simulink model "IMU_Simulation"  (Simulink 7.9)
settings: Solver=FixedStepDiscrete  StartTime=0.0  StopTime=25  FixedStep=.001  RelTol=1e-3
PreLoadFcn:
  | Script_Kalman
values from neighbouring files (symbols this model uses):
  Az = [1 -Ts ;0 1]    [Script_Kalman.m]
  Kz = 1e-3*[.4 ; -.04]    [Script_Kalman.m]
  Ts = .001    (= 0.001)    [Script_Kalman.m]
undefined symbols (not defined in the file or in its folder): dend, DiscIntNeverNeededParam, gaind, numd, polesd, zerosd
libraries: simulink x38
(part 1 of 2)
settings Model: Creator=Lubin  LastModifiedBy=denis.pretre
settings OptimizationCC: InitFltsAndDblsToZero=on
settings DebuggingCC: MultiTaskCondExecSysMsg=warning  MultiTaskRateTransMsg=warning  FcnCallInpInsideContextMsg=Use local settings  StrictBusMsg=Warning
settings HardwareCC: TargetHWDeviceType=32-bit Generic
settings GRTTargetCC: TargetFcnLib=ansi_tfl_tmw.mat  CombineOutputUpdateFcns=off  GRTInterface=on

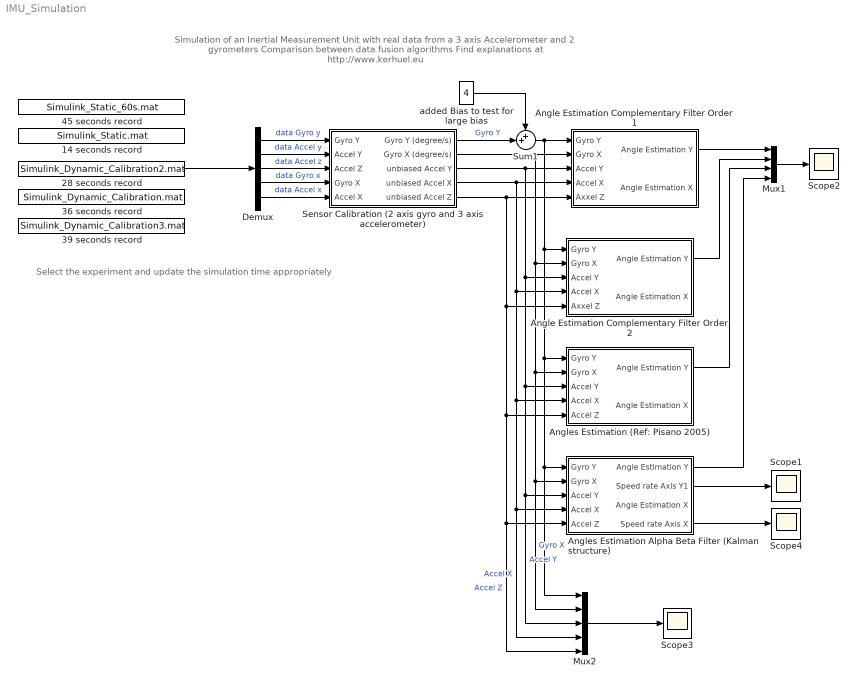
== system IMU_Simulation ==
  note: Simulation of an Inertial Measurement Unit with real data from a 3 axis Accelerometer and 2 gyrometers
      | Comparison between data fusion algorithms
      | Find explanations at http://www.kerhuel.eu
  note: Select the experiment and
      | update the simulation time appropriately
  14 seconds record : FromFile  FileName=Simulink_Static.mat  SampleTime=.001
  28 seconds record : FromFile  FileName=Simulink_Dynamic_Calibration2.mat  SampleTime=.001
  36 seconds record : FromFile  FileName=Simulink_Dynamic_Calibration.mat  SampleTime=.001
  39 seconds record : FromFile  FileName=Simulink_Dynamic_Calibration3.mat  SampleTime=.001
  45 seconds record : FromFile  FileName=Simulink_Static_60s.mat  SampleTime=.001
  Angle Estimation Complementary Filter Order 1 : Subsystem
  Angle Estimation Complementary Filter Order 2 : Subsystem
  Angles Estimation (Ref: Pisano 2005) : Subsystem
  Angles Estimation Alpha Beta Filter (Kalman structure) : Subsystem
  Demux : Demux  Outputs=5
  Mux1 : Mux
  Mux2 : Mux  Inputs=5
  Scope{1..4} (4 alike) : Scope
      Scope1 settings: TimeRange=9.424342105263159  YMin=-7  YMax=7  SaveName=ScopeData3
      Scope2 settings: TickLabels=on  ShowLegends=on  TimeRange=30  YMin=0.5  YMax=10  SaveName=ScopeData4  MaxDataPoints=50000  Decimation=10
      Scope3 settings: TickLabels=on  ShowLegends=on  TimeRange=30  YMin=0.5  YMax=10  SaveName=ScopeData5  MaxDataPoints=50000  Decimation=10
      Scope4 settings: TimeRange=9.424342105263159  YMin=-1.75  YMax=1.75  SaveName=ScopeData6
  Sensor Calibration (2 axis gyro and 3 axis accelerometer) : Subsystem
  Sum1 : Sum  Inputs=++|
  added Bias to test for large bias : Constant  Value=4
  wires:
  Demux/2 -> Sensor Calibration (2 axis gyro and 3 axis accelerometer)/2(Accel Y)  "data Accel y"
  Demux/3 -> Sensor Calibration (2 axis gyro and 3 axis accelerometer)/3(Accel Z)  "data Accel z"
  Demux/4 -> Sensor Calibration (2 axis gyro and 3 axis accelerometer)/4(Gyro X)  "data Gyro x"
  Demux/5 -> Sensor Calibration (2 axis gyro and 3 axis accelerometer)/5(Accel X)  "data Accel x"
  Demux/1 -> Sensor Calibration (2 axis gyro and 3 axis accelerometer)/1(Gyro Y)  "data Gyro y"
  Sensor Calibration (2 axis gyro and 3 axis accelerometer)/1(Gyro Y (degree/s)) -> Sum1/2  "Gyro Y"
  Sensor Calibration (2 axis gyro and 3 axis accelerometer)/2(Gyro X (degree/s)) -> Angle Estimation Complementary Filter Order 1/2(Gyro X), Angles Estimation (Ref: Pisano 2005)/2(Gyro X), Angles Estimation Alpha Beta Filter (Kalman structure)/2(Gyro X), Mux2/2, Angle Estimation Complementary Filter Order 2/2(Gyro X)  "Gyro X"
  Sensor Calibration (2 axis gyro and 3 axis accelerometer)/3(unbiased Accel Y) -> Angle Estimation Complementary Filter Order 1/3(Accel Y), Angles Estimation (Ref: Pisano 2005)/3(Accel Y), Angles Estimation Alpha Beta Filter (Kalman structure)/3(Accel Y), Mux2/3, Angle Estimation Complementary Filter Order 2/3(Accel Y)  "Accel Y"
  Sensor Calibration (2 axis gyro and 3 axis accelerometer)/4(unbiased Accel X) -> Angle Estimation Complementary Filter Order 1/4(Accel X), Angles Estimation (Ref: Pisano 2005)/4(Accel X), Angles Estimation Alpha Beta Filter (Kalman structure)/4(Accel X), Mux2/4, Angle Estimation Complementary Filter Order 2/4(Accel X)  "Accel X"
  Sensor Calibration (2 axis gyro and 3 axis accelerometer)/5(unbiased Accel Z) -> Angle Estimation Complementary Filter Order 1/5(Axxel Z), Angles Estimation (Ref: Pisano 2005)/5(Accel Z), Angles Estimation Alpha Beta Filter (Kalman structure)/5(Accel Z), Mux2/5, Angle Estimation Complementary Filter Order 2/5(Axxel Z)  "Accel Z"
  Mux1/1 -> Scope2/1
  Angle Estimation Complementary Filter Order 1/1(Angle Estimation Y) -> Mux1/1
  Angle Estimation Complementary Filter Order 2/1(Angle Estimation Y) -> Mux1/2
  Angles Estimation (Ref: Pisano 2005)/1(Angle Estimation Y) -> Mux1/3
  Angles Estimation Alpha Beta Filter (Kalman structure)/1(Angle Estimation Y) -> Mux1/4
  Sum1/1 -> Angle Estimation Complementary Filter Order 1/1("Gyro Y "), Angles Estimation (Ref: Pisano 2005)/1(Gyro Y), Angles Estimation Alpha Beta Filter (Kalman structure)/1(Gyro Y), Mux2/1, Angle Estimation Complementary Filter Order 2/1("Gyro Y ")
  added Bias to test for large bias/1 -> Sum1/1
  Angles Estimation Alpha Beta Filter (Kalman structure)/2(Speed rate Axis Y1) -> Scope1/1
  Angles Estimation Alpha Beta Filter (Kalman structure)/4(Speed rate Axis X) -> Scope4/1
  28 seconds record/1 -> Demux/1
  Mux2/1 -> Scope3/1

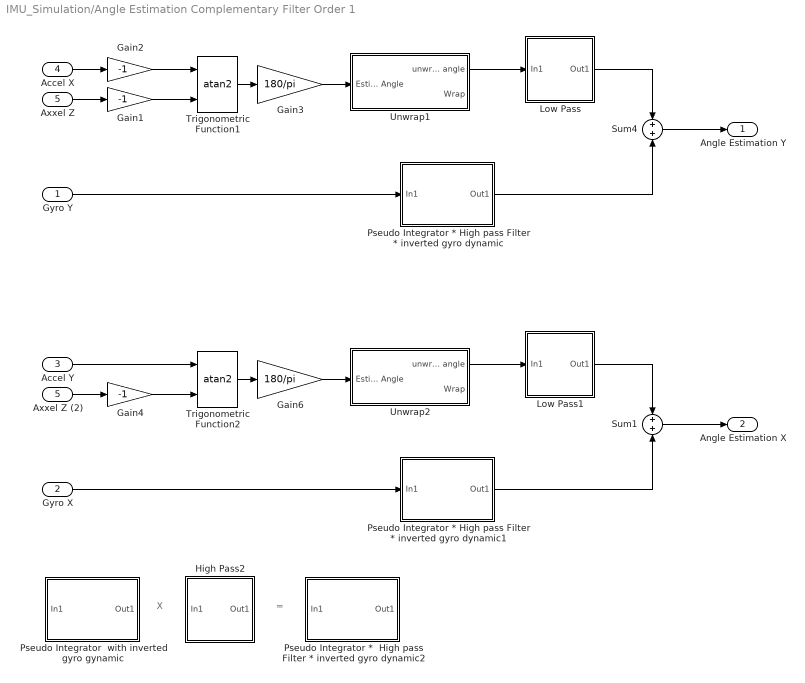
== system IMU_Simulation/Angle Estimation Complementary Filter Order 1 ==
  note: X
  note: =
  "Gyro Y " : Inport
  Gyro X : Inport  Port=2
  Accel Y : Inport  Port=3
  Accel X : Inport  Port=4
  Axxel Z : Inport  Port=5
  Axxel Z (2) : InportShadow  Port=5
  Gain1 : Gain  Gain=-1
  Gain2 : Gain  Gain=-1
  Gain3 : Gain  Gain=180/pi  OutDataTypeStr=float('double')
  Gain4 : Gain  Gain=-1
  Gain6 : Gain  Gain=180/pi  OutDataTypeStr=float('double')
  High Pass2 : Subsystem  mask(DiscretizedZeroPole){Zeros=[0], Poles=[-.5], Gain=1, AbsTol=auto, SampleTime=.001, method=tustin, Wc=1}
      mask prompts: Zeros "Zeros (enter in s-main:)"; Poles "Poles (enter in s-domain:)"; Gain "Gain (enter in s-domain:)"; AbsTol "Absolute tolerance:"; SampleTime "Sample time:"; Wc "Critical Frequency (Hz):"
      mask help: Continuous mask uses c2d to transform parameters onto the Discrete Zero-Pole block inside.
      mask init:
      | st=SampleTime;
      | if length(st)>1
      |     st=SampleTime(1);
      | end
      | if(st>0)
      |     [zerosd,polesd,gaind] = sldiscutil('disczpk', {st,method,Wc,Zeros,Poles,Gain});
      | end	
      | s = get_param(gcb,'maskvalues');
      | zeross = s{1};
      | poless = s{2};
      | gainss = s{3};
      | %zerosc = eval(zeross);
      | %polesc = eval(poless);
      | %gainsc = eval(gainss);
      | sldiscutil('initzpkmask', st);
      | if(st==0)
      | set_param([gcb '/Zero Pole'], 'AbsoluteTolerance', AbsTol);
      | end
      mask StyleString: edit,edit,edit,edit,edit,popup(zoh|foh|tustin|prewarp|matched),edit
      mask CallbackString: |||||hidecrit|
      mask Display:
      | droots(zeross,poless,gainss)
      | text( 0.5, 1.0, method, 'verticalAlignment','top')
  Low Pass : Subsystem  mask(DiscretizedZeroPole){Zeros=[], Poles=[-.5], Gain=.5, AbsTol=auto, SampleTime=.001, method=tustin, Wc=1}
      mask prompts: Zeros "Zeros (enter in s-main:)"; Poles "Poles (enter in s-domain:)"; Gain "Gain (enter in s-domain:)"; AbsTol "Absolute tolerance:"; SampleTime "Sample time:"; Wc "Critical Frequency (Hz):"
      mask help: Continuous mask uses c2d to transform parameters onto the Discrete Zero-Pole block inside.
      mask init: same as IMU_Simulation/Angle Estimation Complementary Filter Order 1/High Pass2
      mask StyleString: edit,edit,edit,edit,edit,popup(zoh|foh|tustin|prewarp|matched),edit
      mask CallbackString: |||||hidecrit|
      mask Display:
      | droots(zeross,poless,gainss)
      | text( 0.5, 1.0, method, 'verticalAlignment','top')
  Low Pass1 : Subsystem  mask(DiscretizedZeroPole){Zeros=[], Poles=[-.5], Gain=.5, AbsTol=auto, SampleTime=.001, method=tustin, Wc=1}
      mask prompts: Zeros "Zeros (enter in s-main:)"; Poles "Poles (enter in s-domain:)"; Gain "Gain (enter in s-domain:)"; AbsTol "Absolute tolerance:"; SampleTime "Sample time:"; Wc "Critical Frequency (Hz):"
      mask help: Continuous mask uses c2d to transform parameters onto the Discrete Zero-Pole block inside.
      mask init: same as IMU_Simulation/Angle Estimation Complementary Filter Order 1/High Pass2
      mask StyleString: edit,edit,edit,edit,edit,popup(zoh|foh|tustin|prewarp|matched),edit
      mask CallbackString: |||||hidecrit|
      mask Display:
      | droots(zeross,poless,gainss)
      | text( 0.5, 1.0, method, 'verticalAlignment','top')
  Pseudo Integrator  with inverted gyro gynamic : Subsystem  mask(DiscretizedZeroPole){Zeros=[-314], Poles=[0], Gain=(1/314), AbsTol=auto, SampleTime=.001, method=tustin, Wc=1}
      mask prompts: Zeros "Zeros (enter in s-main:)"; Poles "Poles (enter in s-domain:)"; Gain "Gain (enter in s-domain:)"; AbsTol "Absolute tolerance:"; SampleTime "Sample time:"; Wc "Critical Frequency (Hz):"
      mask help: Continuous mask uses c2d to transform parameters onto the Discrete Zero-Pole block inside.
      mask init: same as IMU_Simulation/Angle Estimation Complementary Filter Order 1/High Pass2
      mask StyleString: edit,edit,edit,edit,edit,popup(zoh|foh|tustin|prewarp|matched),edit
      mask CallbackString: |||||hidecrit|
      mask Display:
      | droots(zeross,poless,gainss)
      | text( 0.5, 1.0, method, 'verticalAlignment','top')
  Pseudo Integrator *  High pass Filter * inverted gyro dynamic2 : Subsystem  mask(DiscretizedZeroPole){Zeros=[-314], Poles=[-.5], Gain=(1/314), AbsTol=auto, SampleTime=.001, method=tustin, Wc=1}
      mask prompts: Zeros "Zeros (enter in s-main:)"; Poles "Poles (enter in s-domain:)"; Gain "Gain (enter in s-domain:)"; AbsTol "Absolute tolerance:"; SampleTime "Sample time:"; Wc "Critical Frequency (Hz):"
      mask help: Continuous mask uses c2d to transform parameters onto the Discrete Zero-Pole block inside.
      mask init: same as IMU_Simulation/Angle Estimation Complementary Filter Order 1/High Pass2
      mask StyleString: edit,edit,edit,edit,edit,popup(zoh|foh|tustin|prewarp|matched),edit
      mask CallbackString: |||||hidecrit|
      mask Display:
      | droots(zeross,poless,gainss)
      | text( 0.5, 1.0, method, 'verticalAlignment','top')
  Pseudo Integrator * High pass Filter * inverted gyro dynamic : Subsystem  mask(DiscretizedZeroPole){Zeros=[-314], Poles=[-.5], Gain=(1/314), AbsTol=auto, SampleTime=.001, method=tustin, Wc=1}
      mask prompts: Zeros "Zeros (enter in s-main:)"; Poles "Poles (enter in s-domain:)"; Gain "Gain (enter in s-domain:)"; AbsTol "Absolute tolerance:"; SampleTime "Sample time:"; Wc "Critical Frequency (Hz):"
      mask help: Continuous mask uses c2d to transform parameters onto the Discrete Zero-Pole block inside.
      mask init: same as IMU_Simulation/Angle Estimation Complementary Filter Order 1/High Pass2
      mask StyleString: edit,edit,edit,edit,edit,popup(zoh|foh|tustin|prewarp|matched),edit
      mask CallbackString: |||||hidecrit|
      mask Display:
      | droots(zeross,poless,gainss)
      | text( 0.5, 1.0, method, 'verticalAlignment','top')
  Pseudo Integrator * High pass Filter * inverted gyro dynamic1 : Subsystem  mask(DiscretizedZeroPole){Zeros=[-314], Poles=[-.5], Gain=(1/314), AbsTol=auto, SampleTime=.001, method=tustin, Wc=1}
      mask prompts: Zeros "Zeros (enter in s-main:)"; Poles "Poles (enter in s-domain:)"; Gain "Gain (enter in s-domain:)"; AbsTol "Absolute tolerance:"; SampleTime "Sample time:"; Wc "Critical Frequency (Hz):"
      mask help: Continuous mask uses c2d to transform parameters onto the Discrete Zero-Pole block inside.
      mask init: same as IMU_Simulation/Angle Estimation Complementary Filter Order 1/High Pass2
      mask StyleString: edit,edit,edit,edit,edit,popup(zoh|foh|tustin|prewarp|matched),edit
      mask CallbackString: |||||hidecrit|
      mask Display:
      | droots(zeross,poless,gainss)
      | text( 0.5, 1.0, method, 'verticalAlignment','top')
  Sum1 : Sum  SaturateOnIntegerOverflow=on
  Sum4 : Sum  SaturateOnIntegerOverflow=on
  Trigonometric Function1 : Trigonometry  Operator=atan2  OutputSignalType=real
  Trigonometric Function2 : Trigonometry  Operator=atan2  OutputSignalType=real
  Unwrap1 : Subsystem
  Unwrap2 : Subsystem
  Angle Estimation Y : Outport
  Angle Estimation X : Outport  Port=2
  wires:
  Unwrap2/1(unwrap angle) -> Low Pass1/1(In1)
  Gain6/1 -> Unwrap2/1(Estimated Angle)
  Trigonometric Function2/1 -> Gain6/1
  Gain4/1 -> Trigonometric Function2/2
  Gyro X/1 -> Pseudo Integrator * High pass Filter * inverted gyro dynamic1/1(In1)
  Sum1/1 -> Angle Estimation X/1
  Axxel Z (2)/1 -> Gain4/1
  Accel Y/1 -> Trigonometric Function2/1
  Low Pass1/1(Out1) -> Sum1/1
  Unwrap1/1(unwrap angle) -> Low Pass/1(In1)
  Gain3/1 -> Unwrap1/1(Estimated Angle)
  Trigonometric Function1/1 -> Gain3/1
  Gain1/1 -> Trigonometric Function1/2
  Gain2/1 -> Trigonometric Function1/1
  "Gyro Y "/1 -> Pseudo Integrator * High pass Filter * inverted gyro dynamic/1(In1)
  Sum4/1 -> Angle Estimation Y/1
  Axxel Z/1 -> Gain1/1
  Accel X/1 -> Gain2/1
  Low Pass/1(Out1) -> Sum4/1
  Pseudo Integrator * High pass Filter * inverted gyro dynamic1/1(Out1) -> Sum1/2
  Pseudo Integrator * High pass Filter * inverted gyro dynamic/1(Out1) -> Sum4/2

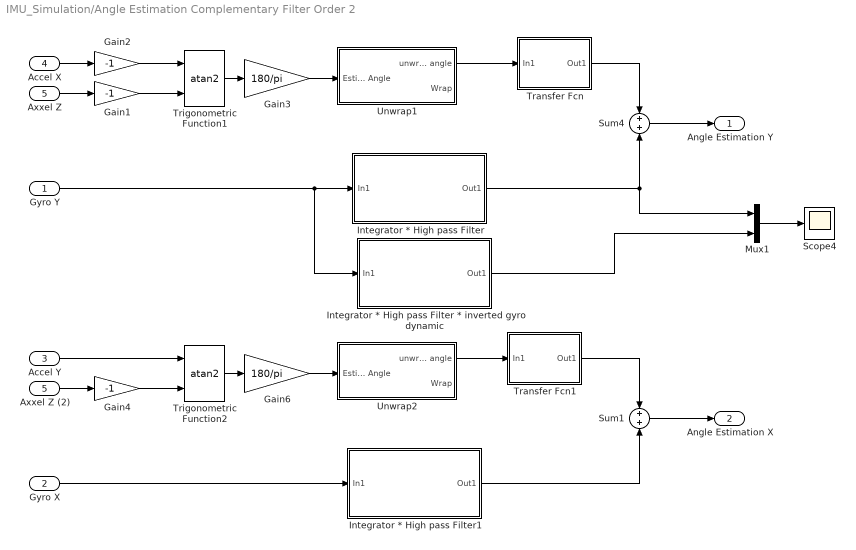
== system IMU_Simulation/Angle Estimation Complementary Filter Order 2 ==
  "Gyro Y " : Inport
  Gyro X : Inport  Port=2
  Accel Y : Inport  Port=3
  Accel X : Inport  Port=4
  Axxel Z : Inport  Port=5
  Axxel Z (2) : InportShadow  Port=5
  Gain1 : Gain  Gain=-1
  Gain2 : Gain  Gain=-1
  Gain3 : Gain  Gain=180/pi  OutDataTypeStr=float('double')
  Gain4 : Gain  Gain=-1
  Gain6 : Gain  Gain=180/pi  OutDataTypeStr=float('double')
  Integrator * High pass Filter : Subsystem  mask(DiscretizedZeroPole){Zeros=[0], Poles=[-.2 -.2], Gain=1, AbsTol=auto, SampleTime=.001, method=tustin, Wc=1}
      mask prompts: Zeros "Zeros (enter in s-main:)"; Poles "Poles (enter in s-domain:)"; Gain "Gain (enter in s-domain:)"; AbsTol "Absolute tolerance:"; SampleTime "Sample time:"; Wc "Critical Frequency (Hz):"
      mask help: Continuous mask uses c2d to transform parameters onto the Discrete Zero-Pole block inside.
      mask init: same as IMU_Simulation/Angle Estimation Complementary Filter Order 1/High Pass2
      mask StyleString: edit,edit,edit,edit,edit,popup(zoh|foh|tustin|prewarp|matched),edit
      mask CallbackString: |||||hidecrit|
      mask Display:
      | droots(zeross,poless,gainss)
      | text( 0.5, 1.0, method, 'verticalAlignment','top')
  Integrator * High pass Filter * inverted gyro dynamic : Subsystem  mask(DiscretizedZeroPole){Zeros=[-314 0], Poles=[-.2 -.2], Gain=(1/314), AbsTol=auto, SampleTime=.001, method=tustin, Wc=1}
      mask prompts: Zeros "Zeros (enter in s-main:)"; Poles "Poles (enter in s-domain:)"; Gain "Gain (enter in s-domain:)"; AbsTol "Absolute tolerance:"; SampleTime "Sample time:"; Wc "Critical Frequency (Hz):"
      mask help: Continuous mask uses c2d to transform parameters onto the Discrete Zero-Pole block inside.
      mask init: same as IMU_Simulation/Angle Estimation Complementary Filter Order 1/High Pass2
      mask StyleString: edit,edit,edit,edit,edit,popup(zoh|foh|tustin|prewarp|matched),edit
      mask CallbackString: |||||hidecrit|
      mask Display:
      | droots(zeross,poless,gainss)
      | text( 0.5, 1.0, method, 'verticalAlignment','top')
  Integrator * High pass Filter1 : Subsystem  mask(DiscretizedZeroPole){Zeros=[0], Poles=[-.2 -.2], Gain=1, AbsTol=auto, SampleTime=.001, method=tustin, Wc=1}
      mask prompts: Zeros "Zeros (enter in s-main:)"; Poles "Poles (enter in s-domain:)"; Gain "Gain (enter in s-domain:)"; AbsTol "Absolute tolerance:"; SampleTime "Sample time:"; Wc "Critical Frequency (Hz):"
      mask help: Continuous mask uses c2d to transform parameters onto the Discrete Zero-Pole block inside.
      mask init: same as IMU_Simulation/Angle Estimation Complementary Filter Order 1/High Pass2
      mask StyleString: edit,edit,edit,edit,edit,popup(zoh|foh|tustin|prewarp|matched),edit
      mask CallbackString: |||||hidecrit|
      mask Display:
      | droots(zeross,poless,gainss)
      | text( 0.5, 1.0, method, 'verticalAlignment','top')
  Mux1 : Mux  Inputs=2
  Scope4 : Scope
      settings: TimeRange=9.424342105263159  YMin=0.5  YMax=6.25  SaveName=ScopeData2  Decimation=10
  Sum1 : Sum  SaturateOnIntegerOverflow=on
  Sum4 : Sum  SaturateOnIntegerOverflow=on
  Transfer Fcn : Subsystem  mask(DiscretizedTransferFcn){Numerator=[.4 .02], Denominator=[1 .4 .02], AbsTol=auto, SampleTime=.001, method=tustin, Wc=0}
      mask prompts: Numerator "Numerator (enter in s-domain:)"; Denominator "Denominator (enter in s-domain:)"; AbsTol "Absolute tolerance:"; SampleTime "Sample time:"; Wc "Critical Frequency (Hz):"
      mask help: Continuous mask uses c2d to transform parameters onto the Discrete Transfer function block inside.
      mask init:
      | st=SampleTime;
      | if length(st)>1
      |     st=SampleTime(1);
      | end
      | if(st>0)
      |     [numd,dend] = sldiscutil('disctransferfcn',{st,method,Wc,Numerator,Denominator});
      | end	
      | s = get_param(gcb,'maskvalues');
      | nums = s{1};
      | dens = s{2};
      | %numc = eval(nums);
      | %denc = eval(dens);
      | sldiscutil('inittfmask', st);
      | if(st==0)
      | set_param([gcb '/Transfer Fcn'], 'AbsoluteTolerance', AbsTol);
      | end
      mask StyleString: edit,edit,edit,edit,popup(zoh|foh|tustin|prewarp|matched),edit
      mask CallbackString: ||||hidecrit|
      mask Display:
      | dpoly(nums,dens)
      | text( 0.5, 1.0, method, 'verticalAlignment','top')
  Transfer Fcn1 : Subsystem  mask(DiscretizedTransferFcn){Numerator=[.4 .02], Denominator=[1 .4 .02], AbsTol=auto, SampleTime=.001, method=tustin, Wc=0}
      mask prompts: Numerator "Numerator (enter in s-domain:)"; Denominator "Denominator (enter in s-domain:)"; AbsTol "Absolute tolerance:"; SampleTime "Sample time:"; Wc "Critical Frequency (Hz):"
      mask help: Continuous mask uses c2d to transform parameters onto the Discrete Transfer function block inside.
      mask init: same as IMU_Simulation/Angle Estimation Complementary Filter Order 2/Transfer Fcn
      mask StyleString: edit,edit,edit,edit,popup(zoh|foh|tustin|prewarp|matched),edit
      mask CallbackString: ||||hidecrit|
      mask Display:
      | dpoly(nums,dens)
      | text( 0.5, 1.0, method, 'verticalAlignment','top')
  Trigonometric Function1 : Trigonometry  Operator=atan2  OutputSignalType=real
  Trigonometric Function2 : Trigonometry  Operator=atan2  OutputSignalType=real
  Unwrap1 : Subsystem
  Unwrap2 : Subsystem
  Angle Estimation Y : Outport
  Angle Estimation X : Outport  Port=2
  wires:
  Integrator * High pass Filter/1(Out1) -> Sum4/2, Mux1/1
  Integrator * High pass Filter1/1(Out1) -> Sum1/2
  Transfer Fcn/1(Out1) -> Sum4/1
  Accel X/1 -> Gain2/1
  Axxel Z/1 -> Gain1/1
  Sum4/1 -> Angle Estimation Y/1
  "Gyro Y "/1 -> Integrator * High pass Filter/1(In1), Integrator * High pass Filter * inverted gyro dynamic/1(In1)
  Gain2/1 -> Trigonometric Function1/1
  Gain1/1 -> Trigonometric Function1/2
  Trigonometric Function1/1 -> Gain3/1
  Gain3/1 -> Unwrap1/1(Estimated Angle)
  Unwrap1/1(unwrap angle) -> Transfer Fcn/1(In1)
  Transfer Fcn1/1(Out1) -> Sum1/1
  Accel Y/1 -> Trigonometric Function2/1
  Axxel Z (2)/1 -> Gain4/1
  Sum1/1 -> Angle Estimation X/1
  Gyro X/1 -> Integrator * High pass Filter1/1(In1)
  Gain4/1 -> Trigonometric Function2/2
  Trigonometric Function2/1 -> Gain6/1
  Gain6/1 -> Unwrap2/1(Estimated Angle)
  Unwrap2/1(unwrap angle) -> Transfer Fcn1/1(In1)
  Integrator * High pass Filter * inverted gyro dynamic/1(Out1) -> Mux1/2
  Mux1/1 -> Scope4/1

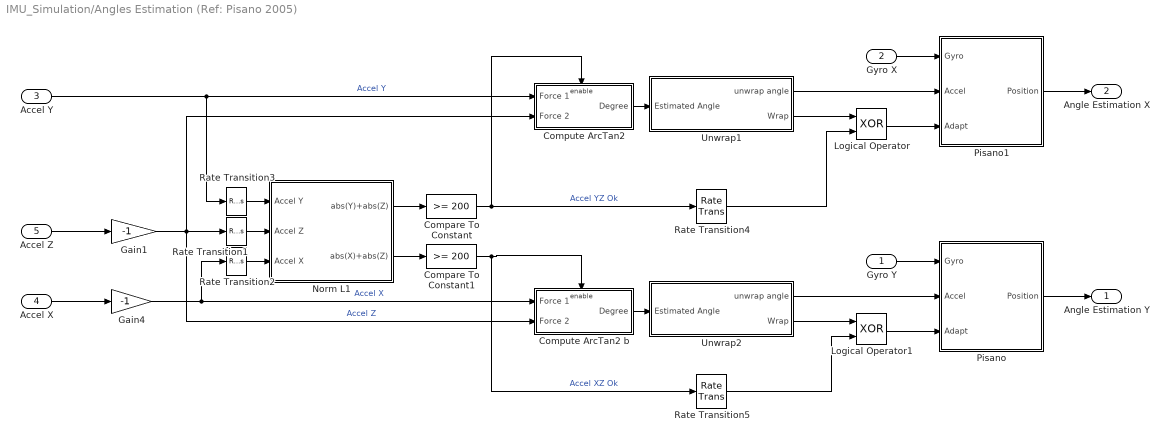
== system IMU_Simulation/Angles Estimation (Ref: Pisano 2005) ==
  Gyro Y : Inport
  Gyro X : Inport  Port=2
  Accel Y : Inport  Port=3
  Accel X : Inport  Port=4
  Accel Z : Inport  Port=5
  Compare To Constant : simulink/Logic and Bit Operations/Compare To Constant  relop=>=  const=200  OutDataTypeStr=boolean  ZeroCross=off
  Compare To Constant1 : simulink/Logic and Bit Operations/Compare To Constant  relop=>=  const=200  OutDataTypeStr=boolean  ZeroCross=off
  Compute ArcTan2 : Subsystem
  Compute ArcTan2 b : Subsystem
  Gain1 : Gain  Gain=-1
  Gain4 : Gain  Gain=-1
  Logical Operator : Logic  Operator=XOR  AllPortsSameDT=off  OutDataTypeStr=boolean
  Logical Operator1 : Logic  Operator=XOR  AllPortsSameDT=off  OutDataTypeStr=boolean
  Norm L1 : Subsystem
  Pisano : Subsystem
  Pisano1 : Subsystem
  Rate Transition1 : RateTransition  Integrity=off  OutPortSampleTime=.2
  Rate Transition2 : RateTransition  Integrity=off  OutPortSampleTime=.2
  Rate Transition3 : RateTransition  Integrity=off  OutPortSampleTime=.2
  Rate Transition4 : RateTransition  Integrity=off  OutPortSampleTime=.001
  Rate Transition5 : RateTransition  Integrity=off  OutPortSampleTime=.001
  Unwrap1 : Subsystem
  Unwrap2 : Subsystem
  Angle Estimation Y : Outport
  Angle Estimation X : Outport  Port=2
  wires:
  Pisano/1(Position) -> Angle Estimation Y/1
  Unwrap2/1(unwrap angle) -> Pisano/2(Accel)
  Unwrap2/2(Wrap) -> Logical Operator1/1
  Logical Operator/1 -> Pisano1/3(Adapt)
  Rate Transition5/1 -> Logical Operator1/2
  Gain1/1 -> Rate Transition1/1, Compute ArcTan2/2(Force 2), Compute ArcTan2 b/2(Force 2)  "Accel Z"
  Logical Operator1/1 -> Pisano/3(Adapt)
  Rate Transition4/1 -> Logical Operator/2
  Unwrap1/2(Wrap) -> Logical Operator/1
  Unwrap1/1(unwrap angle) -> Pisano1/2(Accel)
  Rate Transition3/1 -> Norm L1/1(Accel Y)
  Rate Transition2/1 -> Norm L1/3(Accel X)
  Rate Transition1/1 -> Norm L1/2(Accel Z)
  Compare To Constant1/1 -> Rate Transition5/1, Compute ArcTan2 b/Enable  "Accel XZ Ok"
  Compare To Constant/1 -> Rate Transition4/1, Compute ArcTan2/Enable  "Accel YZ Ok"
  Norm L1/1(abs(Y)+abs(Z)) -> Compare To Constant/1
  Norm L1/2(abs(X)+abs(Z)) -> Compare To Constant1/1
  Accel Z/1 -> Gain1/1
  Gain4/1 -> Rate Transition2/1, Compute ArcTan2 b/1(Force 1)  "Accel X"
  Compute ArcTan2/1(Degree) -> Unwrap1/1(Estimated Angle)
  Compute ArcTan2 b/1(Degree) -> Unwrap2/1(Estimated Angle)
  Accel X/1 -> Gain4/1
  Accel Y/1 -> Compute ArcTan2/1(Force 1), Rate Transition3/1  "Accel Y"
  Gyro X/1 -> Pisano1/1(Gyro)
  Gyro Y/1 -> Pisano/1(Gyro)
  Pisano1/1(Position) -> Angle Estimation X/1

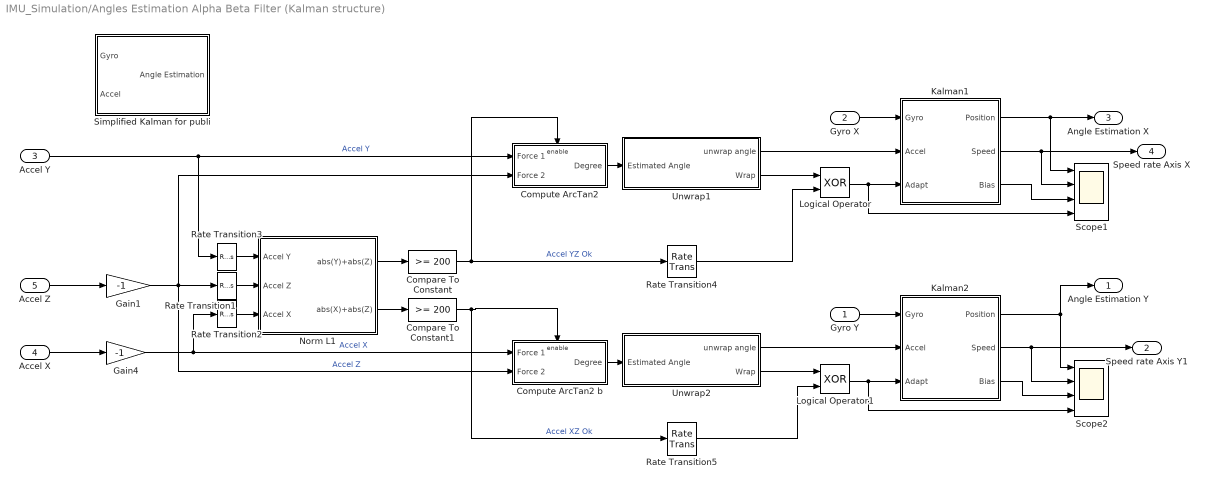
== system IMU_Simulation/Angles Estimation Alpha Beta Filter (Kalman structure) ==
  Gyro Y : Inport
  Gyro X : Inport  Port=2
  Accel Y : Inport  Port=3
  Accel X : Inport  Port=4
  Accel Z : Inport  Port=5
  Compare To Constant : simulink/Logic and Bit Operations/Compare To Constant  relop=>=  const=200  OutDataTypeStr=boolean  ZeroCross=off
  Compare To Constant1 : simulink/Logic and Bit Operations/Compare To Constant  relop=>=  const=200  OutDataTypeStr=boolean  ZeroCross=off
  Compute ArcTan2 : Subsystem
  Compute ArcTan2 b : Subsystem
  Gain1 : Gain  Gain=-1
  Gain4 : Gain  Gain=-1
  Kalman1 : Subsystem
  Kalman2 : Subsystem
  Logical Operator : Logic  Operator=XOR  AllPortsSameDT=off  OutDataTypeStr=boolean
  Logical Operator1 : Logic  Operator=XOR  AllPortsSameDT=off  OutDataTypeStr=boolean
  Norm L1 : Subsystem
  Rate Transition1 : RateTransition  Integrity=off  OutPortSampleTime=.2
  Rate Transition2 : RateTransition  Integrity=off  OutPortSampleTime=.2
  Rate Transition3 : RateTransition  Integrity=off  OutPortSampleTime=.2
  Rate Transition4 : RateTransition  Integrity=off  OutPortSampleTime=.001
  Rate Transition5 : RateTransition  Integrity=off  OutPortSampleTime=.001
  Scope1 : Scope  NumInputPorts=4
      settings: TimeRange=9.424342105263159  YMin=-375~-20~-27.5~0  YMax=-150~40~2.5~1
  Scope2 : Scope  NumInputPorts=4
      settings: TimeRange=9.424342105263159  YMin=-375~-20~-27.5~0  YMax=-150~40~2.5~1
  Simplified Kalman for publi : Subsystem
  Unwrap1 : Subsystem
  Unwrap2 : Subsystem
  Angle Estimation Y : Outport
  Speed rate Axis Y1 : Outport  Port=2
  Angle Estimation X : Outport  Port=3
  Speed rate Axis X : Outport  Port=4
  wires:
  Gyro Y/1 -> Kalman2/1(Gyro)
  Gyro X/1 -> Kalman1/1(Gyro)
  Accel Y/1 -> Rate Transition3/1, Compute ArcTan2/1(Force 1)  "Accel Y"
  Accel X/1 -> Gain4/1
  Compute ArcTan2 b/1(Degree) -> Unwrap2/1(Estimated Angle)
  Compute ArcTan2/1(Degree) -> Unwrap1/1(Estimated Angle)
  Gain4/1 -> Compute ArcTan2 b/1(Force 1), Rate Transition2/1  "Accel X"
  Accel Z/1 -> Gain1/1
  Norm L1/2(abs(X)+abs(Z)) -> Compare To Constant1/1
  Norm L1/1(abs(Y)+abs(Z)) -> Compare To Constant/1
  Compare To Constant/1 -> Compute ArcTan2/Enable, Rate Transition4/1  "Accel YZ Ok"
  Compare To Constant1/1 -> Compute ArcTan2 b/Enable, Rate Transition5/1  "Accel XZ Ok"
  Kalman1/1(Position) -> Angle Estimation X/1, Scope1/1
  Kalman2/1(Position) -> Angle Estimation Y/1, Scope2/1
  Rate Transition1/1 -> Norm L1/2(Accel Z)
  Rate Transition2/1 -> Norm L1/3(Accel X)
  Rate Transition3/1 -> Norm L1/1(Accel Y)
  Unwrap1/1(unwrap angle) -> Kalman1/2(Accel)
  Unwrap1/2(Wrap) -> Logical Operator/1
  Rate Transition4/1 -> Logical Operator/2
  Logical Operator1/1 -> Scope2/4, Kalman2/3(Adapt)
  Gain1/1 -> Compute ArcTan2 b/2(Force 2), Compute ArcTan2/2(Force 2), Rate Transition1/1  "Accel Z"
  Rate Transition5/1 -> Logical Operator1/2
  Logical Operator/1 -> Kalman1/3(Adapt), Scope1/4
  Unwrap2/2(Wrap) -> Logical Operator1/1
  Unwrap2/1(unwrap angle) -> Kalman2/2(Accel)
  Kalman1/2(Speed) -> Scope1/2, Speed rate Axis X/1
  Kalman2/2(Speed) -> Scope2/2, Speed rate Axis Y1/1
  Kalman2/3(Bias) -> Scope2/3
  Kalman1/3(Bias) -> Scope1/3

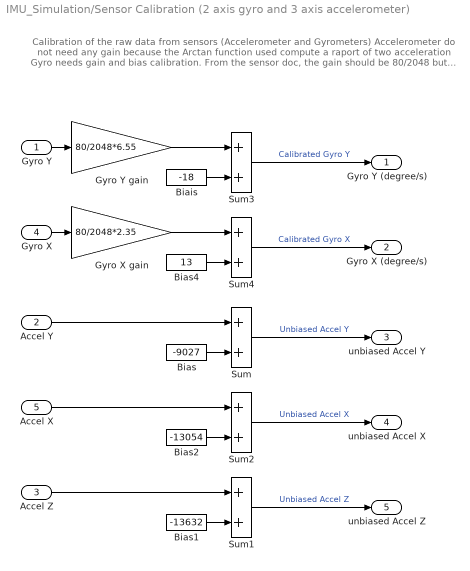
== system IMU_Simulation/Sensor Calibration (2 axis gyro and 3 axis accelerometer) ==
  note: Calibration of the raw data from sensors (Accelerometer and Gyrometers)
      | Accelerometer do not need any gain because the Arctan function used compute a raport of two acceleration
      | Gyro needs gain and bias calibration. From the sensor doc, the gain should be 80/2048 but...
  Gyro Y : Inport
  Accel Y : Inport  Port=2
  Accel Z : Inport  Port=3
  Gyro X : Inport  Port=4
  Accel X : Inport  Port=5
  "Biais " : Constant  Value=-18
  Bias : Constant  Value=-9027
  Bias1 : Constant  Value=-13632
  Bias2 : Constant  Value=-13054
  Bias4 : Constant  Value=13
  Gyro X gain : Gain  Gain=80/2048*2.35  OutDataTypeStr=float('double')
  Gyro Y gain : Gain  Gain=80/2048*6.55  OutDataTypeStr=float('double')
  Sum{,1..4} (5 alike) : Sum
  Gyro Y (degree/s) : Outport
  Gyro X (degree/s) : Outport  Port=2
  unbiased Accel Y : Outport  Port=3
  unbiased Accel X : Outport  Port=4
  unbiased Accel Z : Outport  Port=5
  wires:
  Bias/1 -> Sum/2
  Bias1/1 -> Sum1/2
  Bias2/1 -> Sum2/2
  Gyro Y/1 -> Gyro Y gain/1
  Accel Y/1 -> Sum/1
  Sum/1 -> unbiased Accel Y/1  "Unbiased Accel Y"
  Accel Z/1 -> Sum1/1
  Sum1/1 -> unbiased Accel Z/1  "Unbiased Accel Z"
  Gyro X/1 -> Gyro X gain/1
  Accel X/1 -> Sum2/1
  Sum2/1 -> unbiased Accel X/1  "Unbiased Accel X"
  Gyro Y gain/1 -> Sum3/1
  Sum3/1 -> Gyro Y (degree/s)/1  "Calibrated Gyro Y"
  "Biais "/1 -> Sum3/2
  Gyro X gain/1 -> Sum4/1
  Sum4/1 -> Gyro X (degree/s)/1  "Calibrated Gyro X"
  Bias4/1 -> Sum4/2

== system IMU_Simulation/Angle Estimation Complementary Filter Order 1/High Pass2 ==
  In1 : Inport
  Discrete Zero-Pole : DiscreteZeroPole  Zeros=zerosd  Poles=polesd  Gain=gaind  SampleTime=SampleTime
  Out1 : Outport
  wires:
  Discrete Zero-Pole/1 -> Out1/1
  In1/1 -> Discrete Zero-Pole/1

== system IMU_Simulation/Angle Estimation Complementary Filter Order 1/Low Pass ==
  In1 : Inport
  Discrete Zero-Pole : DiscreteZeroPole  Zeros=zerosd  Poles=polesd  Gain=gaind  SampleTime=SampleTime
  Out1 : Outport
  wires:
  Discrete Zero-Pole/1 -> Out1/1
  In1/1 -> Discrete Zero-Pole/1

== system IMU_Simulation/Angle Estimation Complementary Filter Order 1/Low Pass1 ==
  In1 : Inport
  Discrete Zero-Pole : DiscreteZeroPole  Zeros=zerosd  Poles=polesd  Gain=gaind  SampleTime=SampleTime
  Out1 : Outport
  wires:
  In1/1 -> Discrete Zero-Pole/1
  Discrete Zero-Pole/1 -> Out1/1

== system IMU_Simulation/Angle Estimation Complementary Filter Order 1/Pseudo Integrator  with inverted gyro gynamic ==
  In1 : Inport
  Discrete Zero-Pole : DiscreteZeroPole  Zeros=zerosd  Poles=polesd  Gain=gaind  SampleTime=SampleTime
  Out1 : Outport
  wires:
  Discrete Zero-Pole/1 -> Out1/1
  In1/1 -> Discrete Zero-Pole/1

== system IMU_Simulation/Angle Estimation Complementary Filter Order 1/Pseudo Integrator *  High pass Filter * inverted gyro dynamic2 ==
  In1 : Inport
  Discrete Zero-Pole : DiscreteZeroPole  Zeros=zerosd  Poles=polesd  Gain=gaind  SampleTime=SampleTime
  Out1 : Outport
  wires:
  Discrete Zero-Pole/1 -> Out1/1
  In1/1 -> Discrete Zero-Pole/1

== system IMU_Simulation/Angle Estimation Complementary Filter Order 1/Pseudo Integrator * High pass Filter * inverted gyro dynamic ==
  In1 : Inport
  Discrete Zero-Pole : DiscreteZeroPole  Zeros=zerosd  Poles=polesd  Gain=gaind  SampleTime=SampleTime
  Out1 : Outport
  wires:
  Discrete Zero-Pole/1 -> Out1/1
  In1/1 -> Discrete Zero-Pole/1

== system IMU_Simulation/Angle Estimation Complementary Filter Order 1/Pseudo Integrator * High pass Filter * inverted gyro dynamic1 ==
  In1 : Inport
  Discrete Zero-Pole : DiscreteZeroPole  Zeros=zerosd  Poles=polesd  Gain=gaind  SampleTime=SampleTime
  Out1 : Outport
  wires:
  In1/1 -> Discrete Zero-Pole/1
  Discrete Zero-Pole/1 -> Out1/1

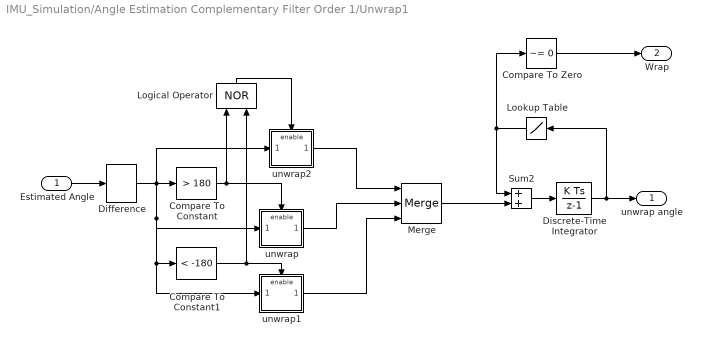
== system IMU_Simulation/Angle Estimation Complementary Filter Order 1/Unwrap1 ==
  Estimated Angle : Inport
  Compare To Constant : simulink/Logic and Bit Operations/Compare To Constant  relop=>  const=180  OutDataTypeStr=uint8  ZeroCross=off
  Compare To Constant1 : simulink/Logic and Bit Operations/Compare To Constant  relop=<  const=-180  OutDataTypeStr=uint8  ZeroCross=off
  Compare To Zero : simulink/Logic and Bit Operations/Compare To Zero  relop=~=  OutDataTypeStr=uint8  ZeroCross=off
  Difference : simulink/Discrete/Difference  ICPrevInput=0.0  InputProcessing=Inherited  OutMin=[]  OutMax=[]  OutDataType=sfix(16)  OutScaling=2^-10  DoSatur=off
  Discrete-Time Integrator : DiscreteIntegrator  gainval=1000  SampleTime=-1  ICPrevOutput=DiscIntNeverNeededParam  ICPrevScaledInput=DiscIntNeverNeededParam
  Logical Operator : Logic  Operator=NOR  AllPortsSameDT=off  OutDataTypeStr=boolean
  Lookup Table : Lookup  InputValues=[-500 -195 195]  Table=[+360 0 -360]  LookUpMeth=Use Input Below
  Merge : Merge  Inputs=3
  Sum2 : Sum
  unwrap : Subsystem  TreatAsAtomicUnit=on
  unwrap1 : Subsystem  TreatAsAtomicUnit=on
  unwrap2 : Subsystem  TreatAsAtomicUnit=on
  unwrap angle : Outport
  Wrap : Outport  Port=2
  wires:
  Discrete-Time Integrator/1 -> unwrap angle/1, Lookup Table/1
  Estimated Angle/1 -> Difference/1
  unwrap1/1(Out1) -> Merge/3
  unwrap/1(Out1) -> Merge/2
  unwrap2/1(Out1) -> Merge/1
  Logical Operator/1 -> unwrap2/Enable
  Compare To Constant1/1 -> Logical Operator/2, unwrap1/Enable
  Compare To Constant/1 -> unwrap/Enable, Logical Operator/1
  Difference/1 -> unwrap2/1(In1), unwrap1/1(In1), Compare To Constant1/1, unwrap/1(In1), Compare To Constant/1
  Sum2/1 -> Discrete-Time Integrator/1
  Merge/1 -> Sum2/2
  Lookup Table/1 -> Sum2/1, Compare To Zero/1
  Compare To Zero/1 -> Wrap/1

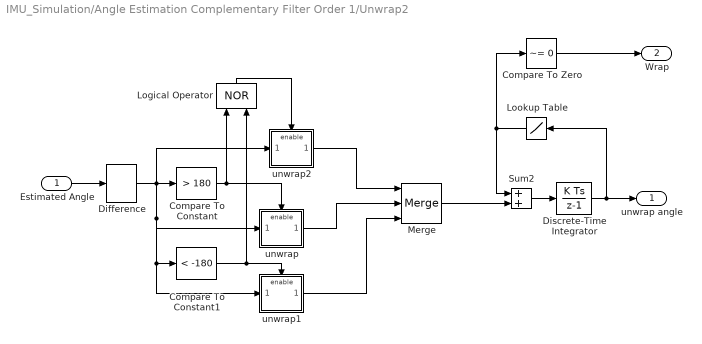
== system IMU_Simulation/Angle Estimation Complementary Filter Order 1/Unwrap2 ==
  Estimated Angle : Inport
  Compare To Constant : simulink/Logic and Bit Operations/Compare To Constant  relop=>  const=180  OutDataTypeStr=uint8  ZeroCross=off
  Compare To Constant1 : simulink/Logic and Bit Operations/Compare To Constant  relop=<  const=-180  OutDataTypeStr=uint8  ZeroCross=off
  Compare To Zero : simulink/Logic and Bit Operations/Compare To Zero  relop=~=  OutDataTypeStr=uint8  ZeroCross=off
  Difference : simulink/Discrete/Difference  ICPrevInput=0.0  InputProcessing=Inherited  OutMin=[]  OutMax=[]  OutDataType=sfix(16)  OutScaling=2^-10  DoSatur=off
  Discrete-Time Integrator : DiscreteIntegrator  gainval=1000  SampleTime=-1  ICPrevOutput=DiscIntNeverNeededParam  ICPrevScaledInput=DiscIntNeverNeededParam
  Logical Operator : Logic  Operator=NOR  AllPortsSameDT=off  OutDataTypeStr=boolean
  Lookup Table : Lookup  InputValues=[-500 -195 195]  Table=[+360 0 -360]  LookUpMeth=Use Input Below
  Merge : Merge  Inputs=3
  Sum2 : Sum
  unwrap : Subsystem  TreatAsAtomicUnit=on
  unwrap1 : Subsystem  TreatAsAtomicUnit=on
  unwrap2 : Subsystem  TreatAsAtomicUnit=on
  unwrap angle : Outport
  Wrap : Outport  Port=2
  wires:
  Compare To Zero/1 -> Wrap/1
  Lookup Table/1 -> Compare To Zero/1, Sum2/1
  Merge/1 -> Sum2/2
  Sum2/1 -> Discrete-Time Integrator/1
  Difference/1 -> Compare To Constant/1, unwrap/1(In1), Compare To Constant1/1, unwrap1/1(In1), unwrap2/1(In1)
  Compare To Constant/1 -> Logical Operator/1, unwrap/Enable
  Compare To Constant1/1 -> unwrap1/Enable, Logical Operator/2
  Logical Operator/1 -> unwrap2/Enable
  unwrap2/1(Out1) -> Merge/1
  unwrap/1(Out1) -> Merge/2
  unwrap1/1(Out1) -> Merge/3
  Estimated Angle/1 -> Difference/1
  Discrete-Time Integrator/1 -> Lookup Table/1, unwrap angle/1

== system IMU_Simulation/Angle Estimation Complementary Filter Order 2/Integrator * High pass Filter ==
  In1 : Inport
  Discrete Zero-Pole : DiscreteZeroPole  Zeros=zerosd  Poles=polesd  Gain=gaind  SampleTime=SampleTime
  Out1 : Outport
  wires:
  Discrete Zero-Pole/1 -> Out1/1
  In1/1 -> Discrete Zero-Pole/1

== system IMU_Simulation/Angle Estimation Complementary Filter Order 2/Integrator * High pass Filter * inverted gyro dynamic ==
  In1 : Inport
  Discrete Zero-Pole : DiscreteZeroPole  Zeros=zerosd  Poles=polesd  Gain=gaind  SampleTime=SampleTime
  Out1 : Outport
  wires:
  Discrete Zero-Pole/1 -> Out1/1
  In1/1 -> Discrete Zero-Pole/1

== system IMU_Simulation/Angle Estimation Complementary Filter Order 2/Integrator * High pass Filter1 ==
  In1 : Inport
  Discrete Zero-Pole : DiscreteZeroPole  Zeros=zerosd  Poles=polesd  Gain=gaind  SampleTime=SampleTime
  Out1 : Outport
  wires:
  In1/1 -> Discrete Zero-Pole/1
  Discrete Zero-Pole/1 -> Out1/1

== system IMU_Simulation/Angle Estimation Complementary Filter Order 2/Transfer Fcn ==
  In1 : Inport
  Discrete Transfer Fcn : DiscreteTransferFcn  Numerator=numd  Denominator=dend  SampleTime=SampleTime
  Out1 : Outport
  wires:
  In1/1 -> Discrete Transfer Fcn/1
  Discrete Transfer Fcn/1 -> Out1/1

== system IMU_Simulation/Angle Estimation Complementary Filter Order 2/Transfer Fcn1 ==
  In1 : Inport
  Discrete Transfer Fcn : DiscreteTransferFcn  Numerator=numd  Denominator=dend  SampleTime=SampleTime
  Out1 : Outport
  wires:
  Discrete Transfer Fcn/1 -> Out1/1
  In1/1 -> Discrete Transfer Fcn/1

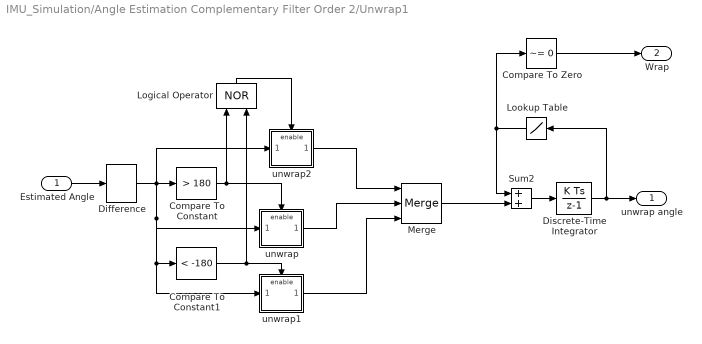
== system IMU_Simulation/Angle Estimation Complementary Filter Order 2/Unwrap1 ==
  Estimated Angle : Inport
  Compare To Constant : simulink/Logic and Bit Operations/Compare To Constant  relop=>  const=180  OutDataTypeStr=uint8  ZeroCross=off
  Compare To Constant1 : simulink/Logic and Bit Operations/Compare To Constant  relop=<  const=-180  OutDataTypeStr=uint8  ZeroCross=off
  Compare To Zero : simulink/Logic and Bit Operations/Compare To Zero  relop=~=  OutDataTypeStr=uint8  ZeroCross=off
  Difference : simulink/Discrete/Difference  ICPrevInput=0.0  InputProcessing=Inherited  OutMin=[]  OutMax=[]  OutDataType=sfix(16)  OutScaling=2^-10  DoSatur=off
  Discrete-Time Integrator : DiscreteIntegrator  gainval=1000  SampleTime=-1  ICPrevOutput=DiscIntNeverNeededParam  ICPrevScaledInput=DiscIntNeverNeededParam
  Logical Operator : Logic  Operator=NOR  AllPortsSameDT=off  OutDataTypeStr=boolean
  Lookup Table : Lookup  InputValues=[-500 -195 195]  Table=[+360 0 -360]  LookUpMeth=Use Input Below
  Merge : Merge  Inputs=3
  Sum2 : Sum
  unwrap : Subsystem  TreatAsAtomicUnit=on
  unwrap1 : Subsystem  TreatAsAtomicUnit=on
  unwrap2 : Subsystem  TreatAsAtomicUnit=on
  unwrap angle : Outport
  Wrap : Outport  Port=2
  wires:
  Compare To Zero/1 -> Wrap/1
  Lookup Table/1 -> Compare To Zero/1, Sum2/1
  Merge/1 -> Sum2/2
  Sum2/1 -> Discrete-Time Integrator/1
  Difference/1 -> Compare To Constant/1, unwrap/1(In1), Compare To Constant1/1, unwrap1/1(In1), unwrap2/1(In1)
  Compare To Constant/1 -> Logical Operator/1, unwrap/Enable
  Compare To Constant1/1 -> unwrap1/Enable, Logical Operator/2
  Logical Operator/1 -> unwrap2/Enable
  unwrap2/1(Out1) -> Merge/1
  unwrap/1(Out1) -> Merge/2
  unwrap1/1(Out1) -> Merge/3
  Estimated Angle/1 -> Difference/1
  Discrete-Time Integrator/1 -> Lookup Table/1, unwrap angle/1

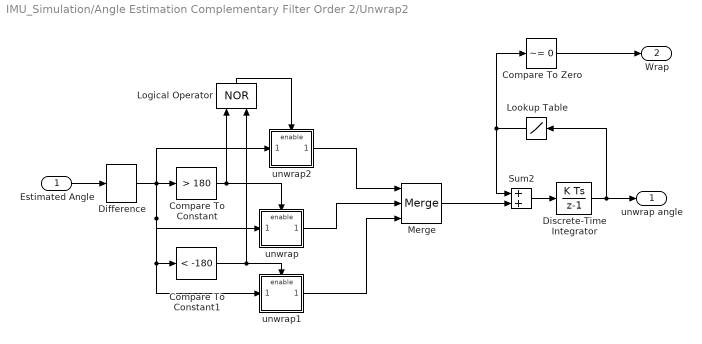
== system IMU_Simulation/Angle Estimation Complementary Filter Order 2/Unwrap2 ==
  Estimated Angle : Inport
  Compare To Constant : simulink/Logic and Bit Operations/Compare To Constant  relop=>  const=180  OutDataTypeStr=uint8  ZeroCross=off
  Compare To Constant1 : simulink/Logic and Bit Operations/Compare To Constant  relop=<  const=-180  OutDataTypeStr=uint8  ZeroCross=off
  Compare To Zero : simulink/Logic and Bit Operations/Compare To Zero  relop=~=  OutDataTypeStr=uint8  ZeroCross=off
  Difference : simulink/Discrete/Difference  ICPrevInput=0.0  InputProcessing=Inherited  OutMin=[]  OutMax=[]  OutDataType=sfix(16)  OutScaling=2^-10  DoSatur=off
  Discrete-Time Integrator : DiscreteIntegrator  gainval=1000  SampleTime=-1  ICPrevOutput=DiscIntNeverNeededParam  ICPrevScaledInput=DiscIntNeverNeededParam
  Logical Operator : Logic  Operator=NOR  AllPortsSameDT=off  OutDataTypeStr=boolean
  Lookup Table : Lookup  InputValues=[-500 -195 195]  Table=[+360 0 -360]  LookUpMeth=Use Input Below
  Merge : Merge  Inputs=3
  Sum2 : Sum
  unwrap : Subsystem  TreatAsAtomicUnit=on
  unwrap1 : Subsystem  TreatAsAtomicUnit=on
  unwrap2 : Subsystem  TreatAsAtomicUnit=on
  unwrap angle : Outport
  Wrap : Outport  Port=2
  wires:
  Discrete-Time Integrator/1 -> unwrap angle/1, Lookup Table/1
  Estimated Angle/1 -> Difference/1
  unwrap1/1(Out1) -> Merge/3
  unwrap/1(Out1) -> Merge/2
  unwrap2/1(Out1) -> Merge/1
  Logical Operator/1 -> unwrap2/Enable
  Compare To Constant1/1 -> Logical Operator/2, unwrap1/Enable
  Compare To Constant/1 -> unwrap/Enable, Logical Operator/1
  Difference/1 -> unwrap2/1(In1), unwrap1/1(In1), Compare To Constant1/1, unwrap/1(In1), Compare To Constant/1
  Sum2/1 -> Discrete-Time Integrator/1
  Merge/1 -> Sum2/2
  Lookup Table/1 -> Sum2/1, Compare To Zero/1
  Compare To Zero/1 -> Wrap/1

== system IMU_Simulation/Angles Estimation (Ref: Pisano 2005)/Compute ArcTan2 ==
  Force 1 : Inport
  Force 2 : Inport  Port=2
  Enable : EnablePort  StatesWhenEnabling=reset
  Gain1 : Gain  Gain=180/pi  OutDataTypeStr=float('double')
  Trigonometric Function1 : Trigonometry  Operator=atan2  OutputSignalType=real
  Degree : Outport
  wires:
  Force 2/1 -> Trigonometric Function1/2
  Force 1/1 -> Trigonometric Function1/1
  Gain1/1 -> Degree/1
  Trigonometric Function1/1 -> Gain1/1

== system IMU_Simulation/Angles Estimation (Ref: Pisano 2005)/Compute ArcTan2 b ==
  Force 1 : Inport
  Force 2 : Inport  Port=2
  Enable : EnablePort  StatesWhenEnabling=reset
  Gain1 : Gain  Gain=180/pi  OutDataTypeStr=float('double')
  Trigonometric Function1 : Trigonometry  Operator=atan2  OutputSignalType=real
  Degree : Outport
  wires:
  Trigonometric Function1/1 -> Gain1/1
  Gain1/1 -> Degree/1
  Force 1/1 -> Trigonometric Function1/1
  Force 2/1 -> Trigonometric Function1/2

== system IMU_Simulation/Angles Estimation (Ref: Pisano 2005)/Norm L1 ==
  Accel Y : Inport
  Accel Z : Inport  Port=2
  Accel X : Inport  Port=3
  Abs : Abs
  Abs1 : Abs
  Abs2 : Abs
  Sum1 : Sum
  Sum3 : Sum
  abs(Y)+abs(Z) : Outport
  abs(X)+abs(Z) : Outport  Port=2
  wires:
  Sum1/1 -> abs(X)+abs(Z)/1
  Accel X/1 -> Abs2/1
  Abs2/1 -> Sum1/2
  Sum3/1 -> abs(Y)+abs(Z)/1
  Accel Z/1 -> Abs1/1
  Accel Y/1 -> Abs/1
  Abs1/1 -> Sum3/2, Sum1/1
  Abs/1 -> Sum3/1

== system IMU_Simulation/Angles Estimation (Ref: Pisano 2005)/Pisano ==
  note: Probleme  du filtrage de l'accelero : dephasage
      | si variation rapide et de forte amplitude, fausse le calcul de l'offset
      | Si on filtre moins, on se prend le biais du aux accelerations
  Gyro : Inport
  Accel : Inport  Port=2
  Adapt : Inport  Port=3
  Constant : Constant  Value=0
  Gain6 : Gain  Gain=1e-3  Multiplication=Matrix(K*u)
  Gain7 : Gain  Gain=Ts  Multiplication=Matrix(K*u)
  Low Pass1 : Subsystem  mask(DiscretizedZeroPole){Zeros=[], Poles=[-30*2*pi], Gain=30*2*pi, AbsTol=auto, SampleTime=.001, method=tustin, Wc=1}
      mask prompts: Zeros "Zeros (enter in s-main:)"; Poles "Poles (enter in s-domain:)"; Gain "Gain (enter in s-domain:)"; AbsTol "Absolute tolerance:"; SampleTime "Sample time:"; Wc "Critical Frequency (Hz):"
      mask help: Continuous mask uses c2d to transform parameters onto the Discrete Zero-Pole block inside.
      mask init: same as IMU_Simulation/Angle Estimation Complementary Filter Order 1/High Pass2
      mask StyleString: edit,edit,edit,edit,edit,popup(zoh|foh|tustin|prewarp|matched),edit
      mask CallbackString: |||||hidecrit|
      mask Display:
      | droots(zeross,poless,gainss)
      | text( 0.5, 1.0, method, 'verticalAlignment','top')
  Multiport Switch : MultiPortSwitch  DataPortOrder=Zero-based contiguous  Inputs=2  zeroidx=on
  Sum2 : Sum  Inputs=++|
  Sum4 : Sum  Inputs=++|
  Sum5 : Sum  Inputs=+-
  Unit Delay2 : UnitDelay  SampleTime=-1
  Position : Outport
  wires:
  Low Pass1/1(Out1) -> Sum5/1
  Unit Delay2/1 -> Sum2/2, Sum5/2
  Gyro/1 -> Gain7/1
  Accel/1 -> Low Pass1/1(In1)
  Gain7/1 -> Sum2/1
  Sum5/1 -> Gain6/1
  Sum2/1 -> Sum4/2
  Multiport Switch/1 -> Sum4/1
  Adapt/1 -> Multiport Switch/1
  Gain6/1 -> Multiport Switch/3
  Constant/1 -> Multiport Switch/2
  Sum4/1 -> Position/1, Unit Delay2/1

== system IMU_Simulation/Angles Estimation (Ref: Pisano 2005)/Pisano1 ==
  note: Probleme  du filtrage de l'accelero : dephasage
      | si variation rapide et de forte amplitude, fausse le calcul de l'offset
      | Si on filtre moins, on se prend le biais du aux accelerations
  Gyro : Inport
  Accel : Inport  Port=2
  Adapt : Inport  Port=3
  Constant : Constant  Value=0
  Gain6 : Gain  Gain=1e-3  Multiplication=Matrix(K*u)
  Gain7 : Gain  Gain=Ts  Multiplication=Matrix(K*u)
  Low Pass1 : Subsystem  mask(DiscretizedZeroPole){Zeros=[], Poles=[-30*2*pi], Gain=30*2*pi, AbsTol=auto, SampleTime=.001, method=tustin, Wc=1}
      mask prompts: Zeros "Zeros (enter in s-main:)"; Poles "Poles (enter in s-domain:)"; Gain "Gain (enter in s-domain:)"; AbsTol "Absolute tolerance:"; SampleTime "Sample time:"; Wc "Critical Frequency (Hz):"
      mask help: Continuous mask uses c2d to transform parameters onto the Discrete Zero-Pole block inside.
      mask init: same as IMU_Simulation/Angle Estimation Complementary Filter Order 1/High Pass2
      mask StyleString: edit,edit,edit,edit,edit,popup(zoh|foh|tustin|prewarp|matched),edit
      mask CallbackString: |||||hidecrit|
      mask Display:
      | droots(zeross,poless,gainss)
      | text( 0.5, 1.0, method, 'verticalAlignment','top')
  Multiport Switch : MultiPortSwitch  DataPortOrder=Zero-based contiguous  Inputs=2  zeroidx=on
  Sum2 : Sum  Inputs=++|
  Sum4 : Sum  Inputs=++|
  Sum5 : Sum  Inputs=+-
  Unit Delay2 : UnitDelay  SampleTime=-1
  Position : Outport
  wires:
  Sum4/1 -> Unit Delay2/1, Position/1
  Constant/1 -> Multiport Switch/2
  Gain6/1 -> Multiport Switch/3
  Adapt/1 -> Multiport Switch/1
  Multiport Switch/1 -> Sum4/1
  Sum2/1 -> Sum4/2
  Sum5/1 -> Gain6/1
  Gain7/1 -> Sum2/1
  Accel/1 -> Low Pass1/1(In1)
  Gyro/1 -> Gain7/1
  Unit Delay2/1 -> Sum5/2, Sum2/2
  Low Pass1/1(Out1) -> Sum5/1

== system IMU_Simulation/Angles Estimation (Ref: Pisano 2005)/Unwrap1 ==
  Estimated Angle : Inport
  Compare To Constant : simulink/Logic and Bit Operations/Compare To Constant  relop=>  const=180  OutDataTypeStr=uint8  ZeroCross=off
  Compare To Constant1 : simulink/Logic and Bit Operations/Compare To Constant  relop=<  const=-180  OutDataTypeStr=uint8  ZeroCross=off
  Compare To Zero : simulink/Logic and Bit Operations/Compare To Zero  relop=~=  OutDataTypeStr=uint8  ZeroCross=off
  Difference : simulink/Discrete/Difference  ICPrevInput=0.0  InputProcessing=Inherited  OutMin=[]  OutMax=[]  OutDataType=sfix(16)  OutScaling=2^-10  DoSatur=off
  Discrete-Time Integrator : DiscreteIntegrator  gainval=1000  SampleTime=-1  ICPrevOutput=DiscIntNeverNeededParam  ICPrevScaledInput=DiscIntNeverNeededParam
  Logical Operator : Logic  Operator=NOR  AllPortsSameDT=off  OutDataTypeStr=boolean
  Lookup Table : Lookup  InputValues=[-500 -195 195]  Table=[+360 0 -360]  LookUpMeth=Use Input Below
  Merge : Merge  Inputs=3
  Sum2 : Sum
  unwrap : Subsystem  TreatAsAtomicUnit=on
  unwrap1 : Subsystem  TreatAsAtomicUnit=on
  unwrap2 : Subsystem  TreatAsAtomicUnit=on
  unwrap angle : Outport
  Wrap : Outport  Port=2
  wires:
  Discrete-Time Integrator/1 -> unwrap angle/1, Lookup Table/1
  Estimated Angle/1 -> Difference/1
  unwrap1/1(Out1) -> Merge/3
  unwrap/1(Out1) -> Merge/2
  unwrap2/1(Out1) -> Merge/1
  Logical Operator/1 -> unwrap2/Enable
  Compare To Constant1/1 -> Logical Operator/2, unwrap1/Enable
  Compare To Constant/1 -> unwrap/Enable, Logical Operator/1
  Difference/1 -> unwrap2/1(In1), unwrap1/1(In1), Compare To Constant1/1, unwrap/1(In1), Compare To Constant/1
  Sum2/1 -> Discrete-Time Integrator/1
  Merge/1 -> Sum2/2
  Lookup Table/1 -> Sum2/1, Compare To Zero/1
  Compare To Zero/1 -> Wrap/1

== system IMU_Simulation/Angles Estimation (Ref: Pisano 2005)/Unwrap2 ==
  Estimated Angle : Inport
  Compare To Constant : simulink/Logic and Bit Operations/Compare To Constant  relop=>  const=180  OutDataTypeStr=uint8  ZeroCross=off
  Compare To Constant1 : simulink/Logic and Bit Operations/Compare To Constant  relop=<  const=-180  OutDataTypeStr=uint8  ZeroCross=off
  Compare To Zero : simulink/Logic and Bit Operations/Compare To Zero  relop=~=  OutDataTypeStr=uint8  ZeroCross=off
  Difference : simulink/Discrete/Difference  ICPrevInput=0.0  InputProcessing=Inherited  OutMin=[]  OutMax=[]  OutDataType=sfix(16)  OutScaling=2^-10  DoSatur=off
  Discrete-Time Integrator : DiscreteIntegrator  gainval=1000  SampleTime=-1  ICPrevOutput=DiscIntNeverNeededParam  ICPrevScaledInput=DiscIntNeverNeededParam
  Logical Operator : Logic  Operator=NOR  AllPortsSameDT=off  OutDataTypeStr=boolean
  Lookup Table : Lookup  InputValues=[-500 -195 195]  Table=[+360 0 -360]  LookUpMeth=Use Input Below
  Merge : Merge  Inputs=3
  Sum2 : Sum
  unwrap : Subsystem  TreatAsAtomicUnit=on
  unwrap1 : Subsystem  TreatAsAtomicUnit=on
  unwrap2 : Subsystem  TreatAsAtomicUnit=on
  unwrap angle : Outport
  Wrap : Outport  Port=2
  wires:
  Compare To Zero/1 -> Wrap/1
  Lookup Table/1 -> Compare To Zero/1, Sum2/1
  Merge/1 -> Sum2/2
  Sum2/1 -> Discrete-Time Integrator/1
  Difference/1 -> Compare To Constant/1, unwrap/1(In1), Compare To Constant1/1, unwrap1/1(In1), unwrap2/1(In1)
  Compare To Constant/1 -> Logical Operator/1, unwrap/Enable
  Compare To Constant1/1 -> unwrap1/Enable, Logical Operator/2
  Logical Operator/1 -> unwrap2/Enable
  unwrap2/1(Out1) -> Merge/1
  unwrap/1(Out1) -> Merge/2
  unwrap1/1(Out1) -> Merge/3
  Estimated Angle/1 -> Difference/1
  Discrete-Time Integrator/1 -> Lookup Table/1, unwrap angle/1

== system IMU_Simulation/Angles Estimation Alpha Beta Filter (Kalman structure)/Compute ArcTan2 ==
  Force 1 : Inport
  Force 2 : Inport  Port=2
  Enable : EnablePort  StatesWhenEnabling=reset
  Gain1 : Gain  Gain=180/pi  OutDataTypeStr=float('double')
  Trigonometric Function1 : Trigonometry  Operator=atan2  OutputSignalType=real
  Degree : Outport
  wires:
  Trigonometric Function1/1 -> Gain1/1
  Gain1/1 -> Degree/1
  Force 1/1 -> Trigonometric Function1/1
  Force 2/1 -> Trigonometric Function1/2

== system IMU_Simulation/Angles Estimation Alpha Beta Filter (Kalman structure)/Compute ArcTan2 b ==
  Force 1 : Inport
  Force 2 : Inport  Port=2
  Enable : EnablePort  StatesWhenEnabling=reset
  Gain1 : Gain  Gain=180/pi  OutDataTypeStr=float('double')
  Trigonometric Function1 : Trigonometry  Operator=atan2  OutputSignalType=real
  Degree : Outport
  wires:
  Force 2/1 -> Trigonometric Function1/2
  Force 1/1 -> Trigonometric Function1/1
  Gain1/1 -> Degree/1
  Trigonometric Function1/1 -> Gain1/1
